simulink library "sdc"  (Simulink 8.1)
settings: Solver=ode1  StartTime=0.0  StopTime=Inf  FixedStep=0.001  RelTol=1e-3
PostLoadFcn:
  | , if any(exist('dsrtsu_mdlpostloadfcn', 'file') == [2, 3, 6]), try dsrtsu_mdlpostloadfcn('Execute', bdroot); catch fprintf('Error in PostLoadFcn (dsrtsu_mdlpostloadfcn) for model "%s":\n %s\n', bdroot, lasterr); end, end,
undefined symbols (not defined in the file or in its folder): ENUM_CAMDYN_ONCOMING, ENUM_CAMDYN_UNDEFINED, ENUM_RADARDYN_ONCOMING, ENUM_RADARDYN_UNDEFINED, KIFO_SameDirecSpeed_kph, ZERO_FLOAT
libraries: hcu_lib x2
settings Model: DSRTSU_INTERNAL_RTI_VER=450  DSRTSU_INTERNAL_RTI_TYPE=rti1401  RTICANMMDATA=struct('GeneralSetupData',struct('modelroot','D:\ELN150201_TAIWAN\trunk\AdasDragon\software\sw_development\arch\app\ifo','generalsettings',struct('filesettings',struct('destfolder',struct('Name','RTICANMM_FILES','Check',1),'buildfolder',struct('Name','.','Check',1),'AbsDestfolder',struct('Name','D:\ELN150201_TAIWAN\trunk\AdasDragon\software\sw_development\arch\app\ifo\RTICANMM_FILES'),'AbsBuildfolder',struct('Name','D:\ELN150201_TAIWAN\trunk\AdasDragon\software\sw_development\arch\app\ifo'))),'options',struct('addpaths',1,'rmpaths',1,'addtrcexclusion',logical(1),'cannavigator',struct('checkmonitoring',0),'show_usrtrc',0,'use_usrtrc',0),'advanced',struct('options',[1 1 1 1 1 1 1 1 1 1 1 1 1 1 1 1 1 1 1 1 1 1 1 1 1 1 1 1 1 1 1 1 1 1 1 1 1 1 1 1 1 1 1 1 1 1 1 1 1 1 1 1 1 1 1 1 1 1 1 1 1 1 1 1 1 1 1 1 1 1 1 1 1 1 1 1 1 1 1 1 1 1 1 1 1 1 1 1 1 1 1 1 1 1 1 1 1 1 1 1]),'MPSetup',{{}},'modelname','sdc','block','sdc'))  DSRTSU_INTERNAL_RTIFPGA=40  Creator=tescamilla  LastModifiedBy=AT015555

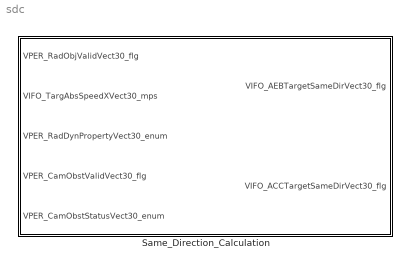
== system sdc ==
  Same_Direction_Calculation : Subsystem

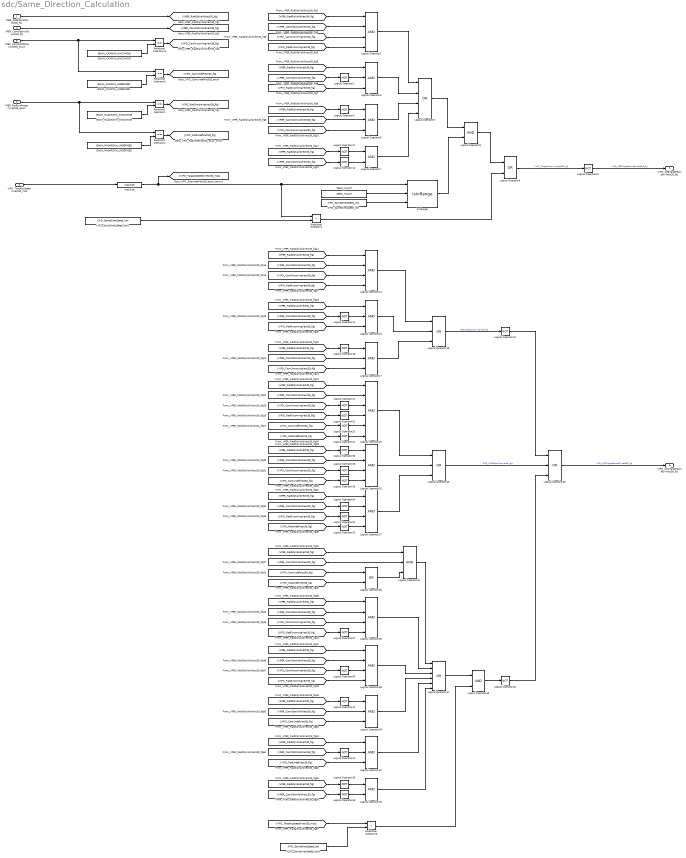
== system sdc/Same_Direction_Calculation ==
  VPER_RadObjValidVect30_flg : Inport
  VIFO_TargAbsSpeedXVect30_mps : Inport  Port=2
  VPER_RadDynPropertyVect30_enum : Inport  Port=3
  VPER_CamObstValidVect30_flg : Inport  Port=4
  VPER_CamObstStatusVect30_enum : Inport  Port=5
  ENUM_CAMDYN_ONCOMING : Constant  Value=ENUM_CAMDYN_ONCOMING
  ENUM_CAMDYN_UNDEFINED : Constant  Value=ENUM_CAMDYN_UNDEFINED
  ENUM_RADARDYN_ONCOMING : Constant  Value=ENUM_RADARDYN_ONCOMING
  ENUM_RADARDYN_UNDEFINED : Constant  Value=ENUM_RADARDYN_UNDEFINED
  IsInRange : hcu_lib/IsInRange  SystemSampleTime=-1
  KIFO_SameDirecSpeed_kph : Constant  Value=KIFO_SameDirecSpeed_kph
  KIFO_SameDirecSpeed_kph1 : Constant  Value=KIFO_SameDirecSpeed_kph
  KIFO_SameDirecSpeed_kph3 : Constant  Value=KIFO_SameDirecSpeed_kph
  Logical Operator{1,13,25,27,36,38} (6 alike) : Logic  Inputs=4  AllPortsSameDT=off  OutDataTypeStr=boolean
  Logical Operator{2,4,10..12,14,16,19,21..24,26,28,30..31,33..34,37,40..41,43..45,48} (25 alike) : Logic  Operator=NOT  AllPortsSameDT=off  OutDataTypeStr=boolean
  Logical Operator{3,5,15,17,32,39,42} (7 alike) : Logic  Inputs=3  AllPortsSameDT=off  OutDataTypeStr=boolean
  Logical Operator18 : Logic  Operator=OR  Inputs=3  AllPortsSameDT=off  OutDataTypeStr=boolean
  Logical Operator20 : Logic  Inputs=6  AllPortsSameDT=off  OutDataTypeStr=boolean
  Logical Operator29 : Logic  Operator=OR  Inputs=3  AllPortsSameDT=off  OutDataTypeStr=boolean
  Logical Operator35 : Logic  Operator=OR  AllPortsSameDT=off  OutDataTypeStr=boolean
  Logical Operator{7..8,46,49} (4 alike) : Logic  AllPortsSameDT=off  OutDataTypeStr=boolean
  Logical Operator47 : Logic  Operator=OR  Inputs=6  AllPortsSameDT=off  OutDataTypeStr=boolean
  Logical Operator50 : Logic  Operator=OR  Inputs=3  AllPortsSameDT=off  OutDataTypeStr=boolean
  Logical Operator6 : Logic  Operator=OR  Inputs=4  AllPortsSameDT=off  OutDataTypeStr=boolean
  Logical Operator9 : Logic  Operator=OR  AllPortsSameDT=off  OutDataTypeStr=boolean
  Relational Operator{1,3..4,11} (4 alike) : RelationalOperator  Operator===  OutDataTypeStr=boolean
  Relational Operator2 : RelationalOperator  Operator=<  OutDataTypeStr=boolean
  Relational Operator5 : RelationalOperator  Operator=<  OutDataTypeStr=boolean
  ZERO_FLOAT : Constant  Value=ZERO_FLOAT
  mps2kph : hcu_lib/mps2kph
  VIFO_AEBTargetSameDirVect30_flg : Outport
  VIFO_ACCTargetSameDirVect30_flg : Outport  Port=2
  wires:
  Logical Operator12/1 -> Logical Operator7/2
  Logical Operator11/1 -> Logical Operator7/1
  Logical Operator9/1 -> Logical Operator10/1  "VIFO_TargetOncomingVect30_flg"
  Logical Operator10/1 -> VIFO_AEBTargetSameDirVect30_flg/1  "VIFO_AEBTargetSameDirVect30_flg"
  Logical Operator8/1 -> Logical Operator9/1
  Relational Operator2/1 -> Logical Operator9/2
  KIFO_SameDirecSpeed_kph1/1 -> Relational Operator2/2
  IsInRange/1 -> Logical Operator8/2
  Logical Operator6/1 -> Logical Operator8/1
  KIFO_SameDirecSpeed_kph/1 -> IsInRange/3
  mps2kph/1 -> [VIFO_TargAbsSpeedXVect30_mps], IsInRange/1, Relational Operator2/1
  ZERO_FLOAT/1 -> IsInRange/2
  VIFO_TargAbsSpeedXVect30_mps/1 -> mps2kph/1
  Logical Operator1/1 -> Logical Operator6/1
  Logical Operator7/1 -> Logical Operator6/4
  Logical Operator5/1 -> Logical Operator6/3
  Logical Operator3/1 -> Logical Operator6/2
  [VPER_RadObjValidVect30_flg] -> Logical Operator11/1
  [VPER_CamObstValidVect30_flg] -> Logical Operator12/1
  Logical Operator4/1 -> Logical Operator5/1
  [VIFO_CamOncomingVect30_flg] -> Logical Operator5/3
  [VPER_CamObstValidVect30_flg] -> Logical Operator5/2
  [VPER_RadObjValidVect30_flg] -> Logical Operator4/1
  [VIFO_RadOncomingVect30_flg] -> Logical Operator3/3
  Logical Operator2/1 -> Logical Operator3/2
  [VPER_CamObstValidVect30_flg] -> Logical Operator2/1
  [VPER_RadObjValidVect30_flg] -> Logical Operator3/1
  ENUM_RADARDYN_ONCOMING/1 -> Relational Operator1/2
  VPER_CamObstStatusVect30_enum/1 -> Relational Operator11/1, Relational Operator3/1
  ENUM_CAMDYN_ONCOMING/1 -> Relational Operator11/2
  [VIFO_RadOncomingVect30_flg] -> Logical Operator1/4
  [VIFO_CamOncomingVect30_flg] -> Logical Operator1/3
  [VPER_CamObstValidVect30_flg] -> Logical Operator1/2
  [VPER_RadObjValidVect30_flg] -> Logical Operator1/1
  Relational Operator1/1 -> [VIFO_RadOncomingVect30_flg]
  Relational Operator11/1 -> [VIFO_CamOncomingVect30_flg]
  VPER_CamObstValidVect30_flg/1 -> [VPER_CamObstValidVect30_flg]
  VPER_RadObjValidVect30_flg/1 -> [VPER_RadObjValidVect30_flg]
  ENUM_CAMDYN_UNDEFINED/1 -> Relational Operator3/2
  Relational Operator3/1 -> [VIFO_CamUndefVect30_flg]
  VPER_RadDynPropertyVect30_enum/1 -> Relational Operator1/1, Relational Operator4/1
  ENUM_RADARDYN_UNDEFINED/1 -> Relational Operator4/2
  Relational Operator4/1 -> [VIFO_RadUndefVect30_flg]
  Logical Operator13/1 -> Logical Operator18/1
  Logical Operator17/1 -> Logical Operator18/3
  Logical Operator15/1 -> Logical Operator18/2
  Logical Operator16/1 -> Logical Operator17/1
  [VIFO_CamOncomingVect30_flg] -> Logical Operator17/3
  [VPER_CamObstValidVect30_flg] -> Logical Operator17/2
  [VPER_RadObjValidVect30_flg] -> Logical Operator16/1
  [VIFO_RadOncomingVect30_flg] -> Logical Operator15/3
  Logical Operator14/1 -> Logical Operator15/2
  [VPER_CamObstValidVect30_flg] -> Logical Operator14/1
  [VPER_RadObjValidVect30_flg] -> Logical Operator15/1
  [VIFO_RadOncomingVect30_flg] -> Logical Operator13/4
  [VIFO_CamOncomingVect30_flg] -> Logical Operator13/3
  [VPER_CamObstValidVect30_flg] -> Logical Operator13/2
  [VPER_RadObjValidVect30_flg] -> Logical Operator13/1
  Logical Operator18/1 -> Logical Operator19/1  "NIFO_ACCOncomingVeh_flg"
  [VIFO_RadOncomingVect30_flg] -> Logical Operator22/1
  [VIFO_CamOncomingVect30_flg] -> Logical Operator21/1
  [VPER_CamObstValidVect30_flg] -> Logical Operator20/2
  [VPER_RadObjValidVect30_flg] -> Logical Operator20/1
  Logical Operator21/1 -> Logical Operator20/3
  Logical Operator22/1 -> Logical Operator20/4
  [VIFO_CamUndefVect30_flg] -> Logical Operator23/1
  Logical Operator23/1 -> Logical Operator20/5
  [VIFO_RadUndefVect30_flg] -> Logical Operator24/1
  Logical Operator24/1 -> Logical Operator20/6
  [VIFO_CamOncomingVect30_flg] -> Logical Operator26/1
  [VPER_CamObstValidVect30_flg] -> Logical Operator25/2
  [VPER_RadObjValidVect30_flg] -> Logical Operator30/1
  Logical Operator26/1 -> Logical Operator25/3
  [VIFO_CamUndefVect30_flg] -> Logical Operator28/1
  Logical Operator28/1 -> Logical Operator25/4
  Logical Operator30/1 -> Logical Operator25/1
  [VIFO_RadOncomingVect30_flg] -> Logical Operator31/1
  [VPER_CamObstValidVect30_flg] -> Logical Operator34/1
  [VPER_RadObjValidVect30_flg] -> Logical Operator27/1
  Logical Operator31/1 -> Logical Operator27/3
  [VIFO_RadUndefVect30_flg] -> Logical Operator33/1
  Logical Operator33/1 -> Logical Operator27/4
  Logical Operator34/1 -> Logical Operator27/2
  Logical Operator20/1 -> Logical Operator29/1
  Logical Operator25/1 -> Logical Operator29/2
  Logical Operator27/1 -> Logical Operator29/3
  Logical Operator35/1 -> Logical Operator32/3
  [VPER_CamObstValidVect30_flg] -> Logical Operator32/2
  [VPER_RadObjValidVect30_flg] -> Logical Operator32/1
  [VIFO_CamUndefVect30_flg] -> Logical Operator35/1
  [VIFO_RadUndefVect30_flg] -> Logical Operator35/2
  [VIFO_RadOncomingVect30_flg] -> Logical Operator37/1
  [VIFO_CamOncomingVect30_flg] -> Logical Operator36/3
  [VPER_CamObstValidVect30_flg] -> Logical Operator36/2
  [VPER_RadObjValidVect30_flg] -> Logical Operator36/1
  Logical Operator37/1 -> Logical Operator36/4
  [VIFO_CamOncomingVect30_flg] -> Logical Operator40/1
  [VPER_CamObstValidVect30_flg] -> Logical Operator38/2
  [VPER_RadObjValidVect30_flg] -> Logical Operator38/1
  [VIFO_RadOncomingVect30_flg] -> Logical Operator38/4
  Logical Operator40/1 -> Logical Operator38/3
  [VIFO_CamUndefVect30_flg] -> Logical Operator39/3
  [VPER_CamObstValidVect30_flg] -> Logical Operator39/2
  [VPER_RadObjValidVect30_flg] -> Logical Operator41/1
  Logical Operator41/1 -> Logical Operator39/1
  [VIFO_RadUndefVect30_flg] -> Logical Operator42/3
  [VPER_CamObstValidVect30_flg] -> Logical Operator44/1
  [VPER_RadObjValidVect30_flg] -> Logical Operator42/1
  Logical Operator44/1 -> Logical Operator42/2
  Logical Operator45/1 -> Logical Operator46/2
  Logical Operator43/1 -> Logical Operator46/1
  [VPER_RadObjValidVect30_flg] -> Logical Operator43/1
  [VPER_CamObstValidVect30_flg] -> Logical Operator45/1
  Logical Operator38/1 -> Logical Operator47/3
  Logical Operator39/1 -> Logical Operator47/4
  Logical Operator36/1 -> Logical Operator47/2
  Logical Operator32/1 -> Logical Operator47/1
  Logical Operator42/1 -> Logical Operator47/5
  Logical Operator46/1 -> Logical Operator47/6
  Logical Operator47/1 -> Logical Operator49/1
  KIFO_SameDirecSpeed_kph3/1 -> Relational Operator5/2
  [VIFO_TargAbsSpeedXVect30_mps] -> Relational Operator5/1
  Relational Operator5/1 -> Logical Operator49/2
  Logical Operator49/1 -> Logical Operator48/1
  Logical Operator29/1 -> Logical Operator50/2  "NIFO_ACCStopOrMoveVeh_flg"
  Logical Operator19/1 -> Logical Operator50/1
  Logical Operator48/1 -> Logical Operator50/3
  Logical Operator50/1 -> VIFO_ACCTargetSameDirVect30_flg/1  "VIFO_ACCTargetSameDirVect30_flg"
